simulink subsystem "logging2workspace"  (R2024b)
settings: Solver=VariableStepAuto  StartTime=0.0  StopTime=10.0  RelTol=1e-3
settings Model: Creator=thesa  LastModifiedBy=thesa
settings RTWCC: GPUComputeCapability=3.5

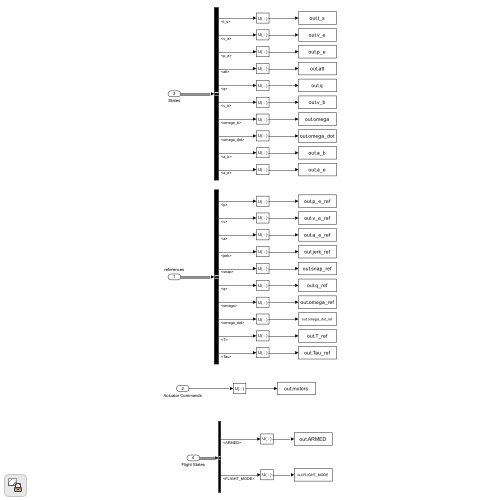
[thumbnail: Simulink's stored preview of the top-level diagram]
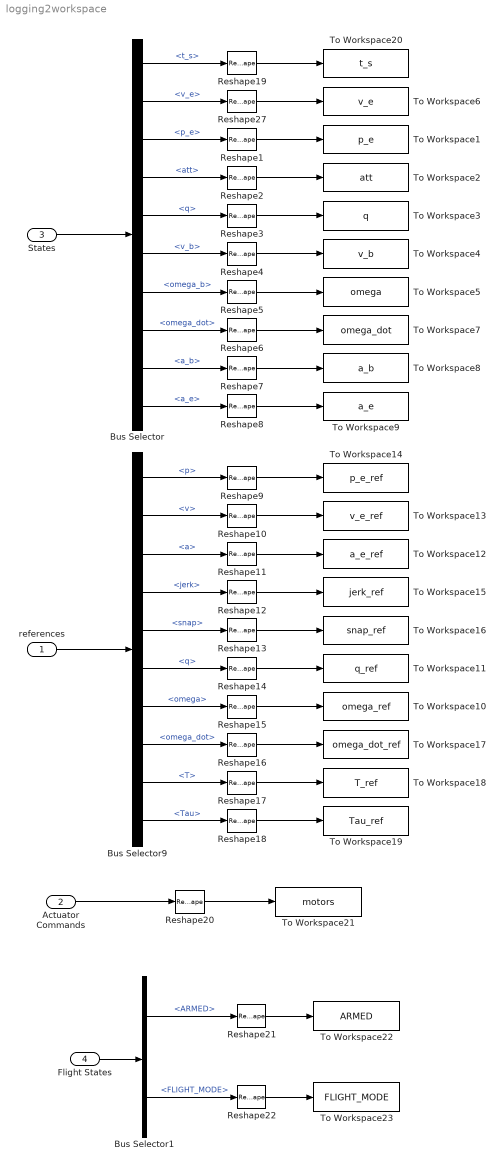
== system logging2workspace ==
  references : Inport
  Actuator Commands : Inport  Port=2
  States : Inport  Port=3
  Flight States : Inport  Port=4
  Bus Selector : BusSelector  OutputSignals=t_s,v_e,p_e,att,q,v_b,omega_b,omega_dot,a_b,a_e
  Bus Selector1 : BusSelector  OutputSignals=ARMED,FLIGHT_MODE
  Bus Selector9 : BusSelector  OutputSignals=trajectory.p,trajectory.v,trajectory.a,trajectory.jerk,trajectory.snap,reconstructed.q,reconstructed.omega,reconstructed.omega_dot,reconstructed.T,reconstructed.Tau
  Reshape{1..22,27} (23 alike) : Reshape
  To Workspace1 : ToWorkspace  VariableName=p_e  SampleTime=-1
  To Workspace10 : ToWorkspace  VariableName=omega_ref  SampleTime=-1
  To Workspace11 : ToWorkspace  VariableName=q_ref  SampleTime=-1
  To Workspace12 : ToWorkspace  VariableName=a_e_ref  SampleTime=-1
  To Workspace13 : ToWorkspace  VariableName=v_e_ref  SampleTime=-1
  To Workspace14 : ToWorkspace  VariableName=p_e_ref  SampleTime=-1
  To Workspace15 : ToWorkspace  VariableName=jerk_ref  SampleTime=-1
  To Workspace16 : ToWorkspace  VariableName=snap_ref  SampleTime=-1
  To Workspace17 : ToWorkspace  VariableName=omega_dot_ref  SampleTime=-1
  To Workspace18 : ToWorkspace  VariableName=T_ref  SampleTime=-1
  To Workspace19 : ToWorkspace  VariableName=Tau_ref  SampleTime=-1
  To Workspace2 : ToWorkspace  VariableName=att  SampleTime=-1
  To Workspace20 : ToWorkspace  VariableName=t_s  SampleTime=-1
  To Workspace21 : ToWorkspace  VariableName=motors  SampleTime=-1
  To Workspace22 : ToWorkspace  VariableName=ARMED  SampleTime=-1
  To Workspace23 : ToWorkspace  VariableName=FLIGHT_MODE  SampleTime=-1
  To Workspace3 : ToWorkspace  VariableName=q  SampleTime=-1
  To Workspace4 : ToWorkspace  VariableName=v_b  SampleTime=-1
  To Workspace5 : ToWorkspace  VariableName=omega  SampleTime=-1
  To Workspace6 : ToWorkspace  VariableName=v_e  SampleTime=-1
  To Workspace7 : ToWorkspace  VariableName=omega_dot  SampleTime=-1
  To Workspace8 : ToWorkspace  VariableName=a_b  SampleTime=-1
  To Workspace9 : ToWorkspace  VariableName=a_e  SampleTime=-1
  wires:
  Reshape18/1 -> To Workspace19/1
  Reshape17/1 -> To Workspace18/1
  Reshape16/1 -> To Workspace17/1
  Reshape13/1 -> To Workspace16/1
  Reshape12/1 -> To Workspace15/1
  Reshape9/1 -> To Workspace14/1
  Reshape10/1 -> To Workspace13/1
  Reshape14/1 -> To Workspace11/1
  Reshape11/1 -> To Workspace12/1
  Reshape15/1 -> To Workspace10/1
  Bus Selector9/10 -> Reshape18/1  "<Tau>"
  Bus Selector9/9 -> Reshape17/1  "<T>"
  Bus Selector9/8 -> Reshape16/1  "<omega_dot>"
  Bus Selector9/7 -> Reshape15/1  "<omega>"
  Bus Selector9/6 -> Reshape14/1  "<q>"
  States/1 -> Bus Selector/1
  references/1 -> Bus Selector9/1
  Bus Selector9/5 -> Reshape13/1  "<snap>"
  Bus Selector9/4 -> Reshape12/1  "<jerk>"
  Bus Selector9/3 -> Reshape11/1  "<a>"
  Bus Selector9/2 -> Reshape10/1  "<v>"
  Bus Selector9/1 -> Reshape9/1  "<p>"
  Reshape8/1 -> To Workspace9/1
  Bus Selector/10 -> Reshape8/1  "<a_e>"
  Reshape7/1 -> To Workspace8/1
  Bus Selector/9 -> Reshape7/1  "<a_b>"
  Reshape6/1 -> To Workspace7/1
  Bus Selector/8 -> Reshape6/1  "<omega_dot>"
  Reshape5/1 -> To Workspace5/1
  Bus Selector/7 -> Reshape5/1  "<omega_b>"
  Reshape4/1 -> To Workspace4/1
  Bus Selector/6 -> Reshape4/1  "<v_b>"
  Bus Selector/5 -> Reshape3/1  "<q>"
  Reshape3/1 -> To Workspace3/1
  Reshape2/1 -> To Workspace2/1
  Bus Selector/4 -> Reshape2/1  "<att>"
  Reshape1/1 -> To Workspace1/1
  Bus Selector/3 -> Reshape1/1  "<p_e>"
  Bus Selector/2 -> Reshape27/1  "<v_e>"
  Reshape27/1 -> To Workspace6/1
  Bus Selector/1 -> Reshape19/1  "<t_s>"
  Reshape19/1 -> To Workspace20/1
  Actuator Commands/1 -> Reshape20/1
  Reshape20/1 -> To Workspace21/1
  Flight States/1 -> Bus Selector1/1
  Bus Selector1/1 -> Reshape21/1  "<ARMED>"
  Bus Selector1/2 -> Reshape22/1  "<FLIGHT_MODE>"
  Reshape21/1 -> To Workspace22/1
  Reshape22/1 -> To Workspace23/1
